simulink model "motorul"  (R2022b)
settings: Solver=VariableStepAuto  StartTime=0.0  StopTime=10.0  RelTol=1e-3
settings Model: Creator=Ruxandra  LastModifiedBy=Ruxandra

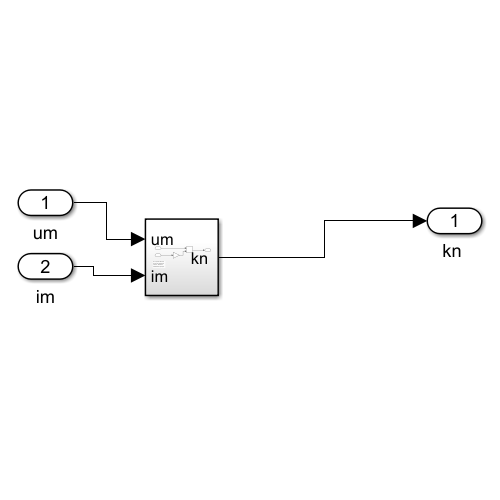
[thumbnail: Simulink's stored preview of the top-level diagram]
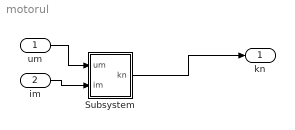
== system motorul ==
  um : Inport
  im : Inport  Port=2
  Subsystem : Subsystem
  "kn " : Outport
  wires:
  um/1 -> Subsystem/1(um)
  im/1 -> Subsystem/2(im)
  Subsystem/1("kn ") -> "kn "/1

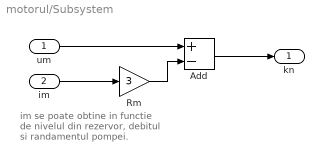
== system motorul/Subsystem ==
  note: im se poate obtine in functie de nivelul din rezervor, debitul si randamentul pompei.
  um : Inport
  im : Inport  Port=2
  Add : Sum  Inputs=+-
  Rm : Gain  Gain=3
  "kn " : Outport
  wires:
  im/1 -> Rm/1
  um/1 -> Add/1
  Rm/1 -> Add/2
  Add/1 -> "kn "/1
